simulink model "UAVmode"  (Simulink 8.3)
settings: Solver=ode45  StartTime=0.0  StopTime=20.0  RelTol=1e-3
values from neighbouring files (symbols this model uses):
  AngKD = UAV.AngKD    [UAVSimStart.m]
  AngKP = UAV.AngKP    [UAVSimStart.m]
  PosKD = UAV.PosKD    [UAVSimStart.m]
  PosKP = UAV.PosKP    [UAVSimStart.m]
  UAV = struct('Is',eye(3),'Is_inv',eye(3),'Mass',10,'L',1,'AllocationMoment',0,'RotorNum',0,'Type',[],'AllocationRotate',0,'GravityAcc',9.81,'Init_Pos',[0,0,0],'Init_Pos_Vel',[0,0,0],           'Course_ANG',0,'RWS',eye(3),'RSW',eye(3),'MaxTargetAng',[0,0,0],'MinTargetAng',[0,0,0],'TargetPos',[0,0,0],'TargetPos_Vel',[0,0,0],'LineTrack_ACC',[0,0,0],'LineTrack_Vel',[0,0,0],'CircleTrc_AngleACC',0.01,'CircleT ...(+517 chars)    [UAVSimStart.m]
libraries: fuzblock x3, simulink x2, aerolibtransform2 x2, vrlib x1
settings Model: Creator=Administrator  LastModifiedBy=jyl58
settings DataIOCC: SignalLoggingSaveFormat=Dataset
settings OptimizationCC: ExpressionDepthLimit=2147483647
settings DebuggingCC: FcnCallInpInsideContextMsg=EnableAllAsWarning
settings GRTTargetCC: CombineOutputUpdateFcns=on  GRTInterface=off

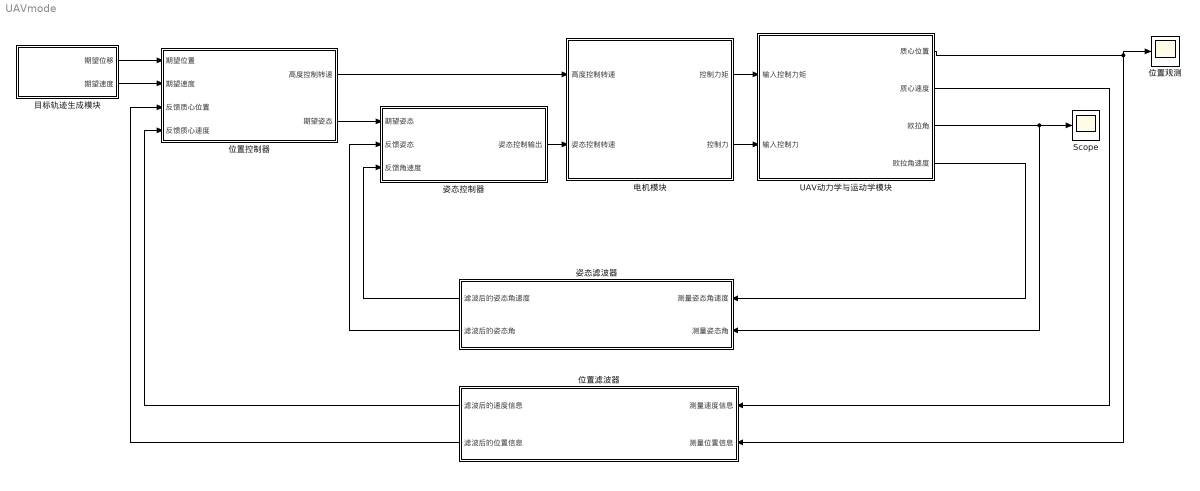
== system UAVmode ==
  Scope : Scope
      settings: YMin=-0.01  YMax=0.15
  UAV动力学与运动学模块 : Subsystem
  位置控制器 : Subsystem
  位置滤波器 : Subsystem
  位置观测 : Scope
      settings: YMin=-0.025  YMax=0.55  SaveName=ScopeData7
  姿态控制器 : Subsystem
  姿态滤波器 : Subsystem
  电机模块 : Subsystem
  目标轨迹生成模块 : Subsystem
  wires:
  电机模块/1(控制力矩) -> UAV动力学与运动学模块/1(输入控制力矩)
  姿态滤波器/2(滤波后的姿态角) -> 姿态控制器/2(反馈姿态)
  姿态滤波器/1(滤波后的姿态角速度) -> 姿态控制器/3(反馈角速度)
  电机模块/2(控制力) -> UAV动力学与运动学模块/2(输入控制力)
  UAV动力学与运动学模块/3(欧拉角) -> Scope/1, 姿态滤波器/2(测量姿态角)
  UAV动力学与运动学模块/4(欧拉角速度) -> 姿态滤波器/1(测量姿态角速度)
  UAV动力学与运动学模块/2(质心速度) -> 位置滤波器/1(测量速度信息)
  位置滤波器/1(滤波后的速度信息) -> 位置控制器/4(反馈质心速度)
  位置滤波器/2(滤波后的位置信息) -> 位置控制器/3(反馈质心位置)
  位置控制器/2(期望姿态) -> 姿态控制器/1(期望姿态)
  姿态控制器/1(姿态控制输出) -> 电机模块/2(姿态控制转速)
  目标轨迹生成模块/1(期望位移) -> 位置控制器/1(期望位置)
  目标轨迹生成模块/2(期望速度) -> 位置控制器/2(期望速度)
  位置控制器/1(高度控制转速) -> 电机模块/1(高度控制转速)
  UAV动力学与运动学模块/1(质心位置) -> 位置滤波器/2(测量位置信息), 位置观测/1

== system UAVmode/UAV动力学与运动学模块 ==
  输入控制力矩 : Inport
  输入控制力 : Inport  Port=2
  Terminator : Terminator
  姿态方程 : Subsystem
  质心运动方程 : Subsystem
  质心位置 : Outport
  质心速度 : Outport  Port=2
  欧拉角 : Outport  Port=3
  欧拉角速度 : Outport  Port=4
  wires:
  输入控制力矩/1 -> 姿态方程/1(控制力矩)
  姿态方程/2(欧拉角) -> 欧拉角/1, 质心运动方程/2(姿态角)
  姿态方程/3(欧拉角速度) -> 欧拉角速度/1
  输入控制力/1 -> 质心运动方程/1(控制力输入)
  质心运动方程/1(惯性系下质心位置) -> 质心位置/1
  质心运动方程/2(惯性系下速度) -> 质心速度/1
  姿态方程/1(惯性加速度) -> Terminator/1

== system UAVmode/位置控制器 ==
  期望位置 : Inport
  期望速度 : Inport  Port=2
  反馈质心位置 : Inport  Port=3
  反馈质心速度 : Inport  Port=4
  位置控制器 : Subsystem
  质心位置信息 : Subsystem
  高度控制转速 : Outport
  期望姿态 : Outport  Port=2
  wires:
  质心位置信息/1(位置偏差) -> 位置控制器/1(质心位置偏差)
  质心位置信息/2(速度偏差) -> 位置控制器/2(速度偏差)
  反馈质心位置/1 -> 质心位置信息/3(反馈质心位置)
  位置控制器/1(高度转速) -> 高度控制转速/1
  位置控制器/2(期望姿态) -> 期望姿态/1
  反馈质心速度/1 -> 质心位置信息/4(反馈质心速度)
  期望位置/1 -> 质心位置信息/1(期望位置)
  期望速度/1 -> 质心位置信息/2(期望速度)

== system UAVmode/位置滤波器 ==
  note: 暂不加滤波器
  note: 暂不加滤波器
  测量速度信息 : Inport
  测量位置信息 : Inport  Port=2
  滤波后的速度信息 : Outport
  滤波后的位置信息 : Outport  Port=2
  wires:
  测量位置信息/1 -> 滤波后的位置信息/1
  测量速度信息/1 -> 滤波后的速度信息/1

== system UAVmode/姿态控制器 ==
  期望姿态 : Inport
  反馈姿态 : Inport  Port=2
  反馈角速度 : Inport  Port=3
  姿态偏差信息 : Subsystem
  姿态控制器 : Subsystem
  期望角速度 : Constant  Value=UAV.TargetAng_Vel
  姿态控制输出 : Outport
  wires:
  反馈姿态/1 -> 姿态偏差信息/2(反馈姿态), 姿态控制器/4(反馈姿态)
  反馈角速度/1 -> 姿态偏差信息/4(反馈角速度), 姿态控制器/3(反馈角速度)
  期望角速度/1 -> 姿态偏差信息/3(期望角速度)
  期望姿态/1 -> 姿态偏差信息/1(期望姿态)
  姿态控制器/1(控制输出) -> 姿态控制输出/1
  姿态偏差信息/1(姿态角偏差) -> 姿态控制器/1(姿态角偏差)
  姿态偏差信息/2(姿态角速度偏差) -> 姿态控制器/2(角速度偏差)

== system UAVmode/姿态滤波器 ==
  note: 暂时不加滤波
  note: 暂时不加滤波
  测量姿态角速度 : Inport
  测量姿态角 : Inport  Port=2
  滤波后的姿态角速度 : Outport
  滤波后的姿态角 : Outport  Port=2
  wires:
  测量姿态角/1 -> 滤波后的姿态角/1
  测量姿态角速度/1 -> 滤波后的姿态角速度/1

== system UAVmode/电机模块 ==
  高度控制转速 : Inport
  姿态控制转速 : Inport  Port=2
  执行 : Subsystem
  转速融合 : Subsystem
  控制力矩 : Outport
  控制力 : Outport  Port=2
  wires:
  执行/1(控制力矩输出) -> 控制力矩/1
  执行/2(控制力输出) -> 控制力/1
  姿态控制转速/1 -> 转速融合/2(姿态控制转速)
  高度控制转速/1 -> 转速融合/1(高度控制转速)
  转速融合/1(电机总控制转速输出) -> 执行/1(控制转速)

== system UAVmode/目标轨迹生成模块 ==
  Constant : Constant  Value=0
  Constant1 : Constant  Value=0
  圆轨迹生成器 : Subsystem
  直线轨迹生成器 : Subsystem
  轨迹类型选择开关 : Constant  Value=UAV.TraceType
  轨迹选择器 : MultiPortSwitch
  轨迹选择器1 : MultiPortSwitch
  期望位移 : Outport
  期望速度 : Outport  Port=2
  wires:
  直线轨迹生成器/1(期望位置) -> 轨迹选择器/2
  圆轨迹生成器/1(期望位置) -> 轨迹选择器/3
  轨迹选择器1/1 -> 期望速度/1
  圆轨迹生成器/2(期望速度) -> 轨迹选择器1/3
  直线轨迹生成器/2(期望速度) -> 轨迹选择器1/2
  轨迹类型选择开关/1 -> 轨迹选择器1/1, 轨迹选择器/1
  Constant/1 -> 轨迹选择器/4
  Constant1/1 -> 轨迹选择器1/4
  轨迹选择器/1 -> 期望位移/1

== system UAVmode/UAV动力学与运动学模块/姿态方程 ==
  控制力矩 : Inport
  Sum : Sum  Inputs=|++
  姿态动力学方程 : Subsystem
  姿态运动学 : Subsystem
  干扰生成模块 : Subsystem
  惯性加速度 : Outport
  欧拉角 : Outport  Port=2
  欧拉角速度 : Outport  Port=3
  wires:
  姿态动力学方程/1(惯性角速度) -> 姿态运动学/1(Wbi), 惯性加速度/1
  姿态运动学/1(欧拉角) -> 欧拉角/1
  姿态运动学/2(欧拉角速度) -> 欧拉角速度/1
  控制力矩/1 -> Sum/1
  Sum/1 -> 姿态动力学方程/1(输入力矩)
  干扰生成模块/1(干扰输出) -> Sum/2

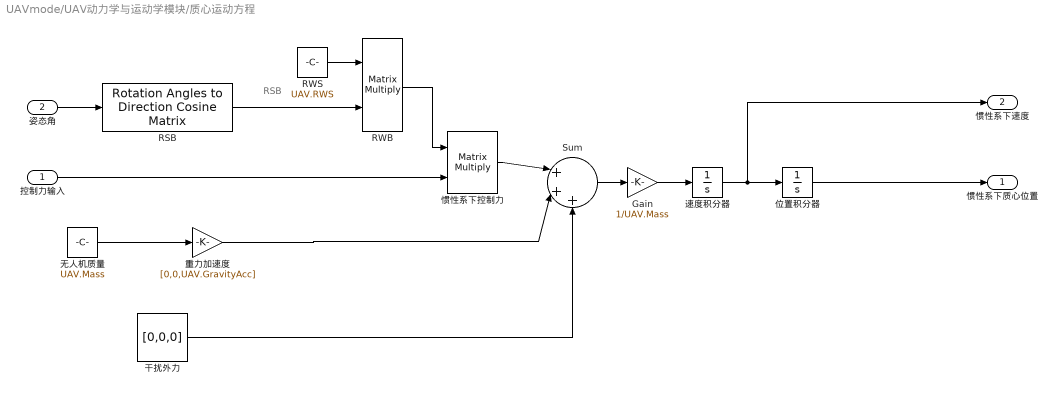
== system UAVmode/UAV动力学与运动学模块/质心运动方程 ==
  note: RSB
  控制力输入 : Inport
  姿态角 : Inport  Port=2
  Gain : Gain  Gain=1/UAV.Mass
  RSB : aerolibtransform2/Rotation Angles to Direction Cosine Matrix  rotationOrder=XYZ
  RWB : Product  Multiplication=Matrix(*)  RndMeth=Zero
  RWS : Constant  Value=UAV.RWS
  Sum : Sum  Inputs=|+++
  位置积分器 : Integrator  InitialCondition=UAV.Init_Pos
  干扰外力 : Constant  Value=[0,0,0]
  惯性系下控制力 : Product  Multiplication=Matrix(*)  RndMeth=Zero
  无人机质量 : Constant  Value=UAV.Mass
  速度积分器 : Integrator  InitialCondition=[0,0,0]
  重力加速度 : Gain  Gain=[0,0,UAV.GravityAcc]
  惯性系下质心位置 : Outport
  惯性系下速度 : Outport  Port=2
  wires:
  无人机质量/1 -> 重力加速度/1
  重力加速度/1 -> Sum/2
  速度积分器/1 -> 位置积分器/1, 惯性系下速度/1
  位置积分器/1 -> 惯性系下质心位置/1
  控制力输入/1 -> 惯性系下控制力/2
  惯性系下控制力/1 -> Sum/1
  干扰外力/1 -> Sum/3
  姿态角/1 -> RSB/1
  RSB/1 -> RWB/2
  RWS/1 -> RWB/1
  RWB/1 -> 惯性系下控制力/1
  Gain/1 -> 速度积分器/1
  Sum/1 -> Gain/1

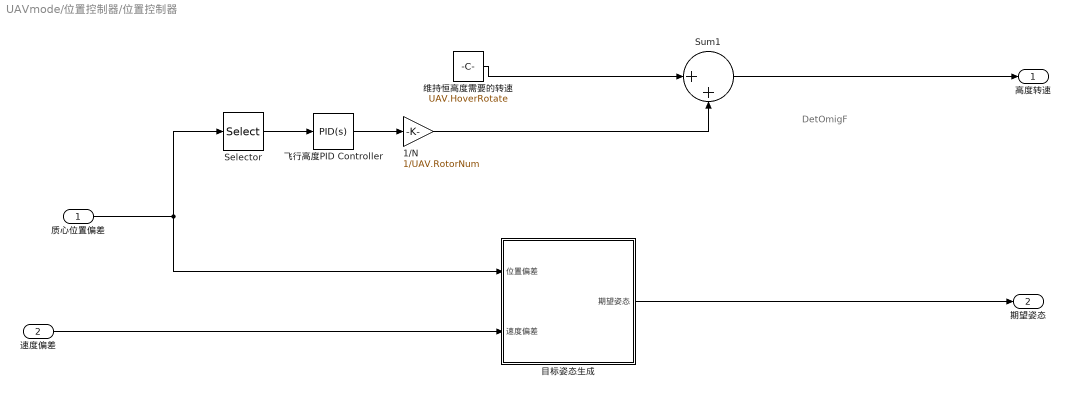
== system UAVmode/位置控制器/位置控制器 ==
  note: DetOmigF
  质心位置偏差 : Inport
  速度偏差 : Inport  Port=2
  1/N : Gain  Gain=1/UAV.RotorNum
  Selector : Selector  InputPortWidth=3  Indices=[3]
  Sum1 : Sum  Inputs=|++
  目标姿态生成 : Subsystem
  维持恒高度需要的转速 : Constant  Value=UAV.HoverRotate
  飞行高度PID Controller : simulink/Continuous/PID Controller  Controller=PID  TimeDomain=Continuous-time  SampleTime=1  IntegratorMethod=Forward Euler  FilterMethod=Forward Euler  Form=Parallel  P=-UAV.AltKP  I=-UAV.AltKI  D=-UAV.AltKD  N=1  InitialConditionSource=internal  InitialConditionForIntegrator=0  InitialConditionForFilter=0  ExternalReset=none  LimitOutput=off  UpperSaturationLimit=inf  LowerSaturationLimit=-inf  LinearizeAsGain=off  AntiWindupMode=none  Kb=1  TrackingMode=off  Kt=1  PParamMin=[]  PParamMax=[]  IParamMin=[]  IParamMax=[]  DParamMin=[]  DParamMax=[]  NParamMin=[]  NParamMax=[]  KbParamMin=[]  KbParamMax=[]  KtParamMin=[]  KtParamMax=[]  POutMin=[]  POutMax=[]  IOutMin=[]  IOutMax=[]  DOutMin=[]  DOutMax=[]  NOutMin=[]  NOutMax=[]  KbOutMin=[]  KbOutMax=[]  KtOutMin=[]  KtOutMax=[]  IntegratorOutMin=[]  IntegratorOutMax=[]  FilterOutMin=[]  FilterOutMax=[]  SumOutMin=[]  SumOutMax=[]  SumI1OutMin=[]  SumI1OutMax=[]  SumI2OutMin=[]  SumI2OutMax=[]  SumI3OutMin=[]  SumI3OutMax=[]  SumDOutMin=[]  SumDOutMax=[]  SaturationOutMin=[]  SaturationOutMax=[]  IntegratorContinuousStateAttributes=''  IntegratorStateMustResolveToSignalObject=off  IntegratorRTWStateStorageClass=Auto  FilterContinuousStateAttributes=''  FilterStateMustResolveToSignalObject=off  FilterRTWStateStorageClass=Auto
  高度转速 : Outport
  期望姿态 : Outport  Port=2
  wires:
  目标姿态生成/1(期望姿态) -> 期望姿态/1
  Sum1/1 -> 高度转速/1
  维持恒高度需要的转速/1 -> Sum1/1
  质心位置偏差/1 -> 目标姿态生成/1(位置偏差), Selector/1
  速度偏差/1 -> 目标姿态生成/2(速度偏差)
  飞行高度PID Controller/1 -> 1/N/1
  1/N/1 -> Sum1/2
  Selector/1 -> 飞行高度PID Controller/1

== system UAVmode/位置控制器/质心位置信息 ==
  期望位置 : Inport
  期望速度 : Inport  Port=2
  反馈质心位置 : Inport  Port=3
  反馈质心速度 : Inport  Port=4
  Sum : Sum  Inputs=|+-
  Sum1 : Sum  Inputs=|+-
  位置偏差 : Outport
  速度偏差 : Outport  Port=2
  wires:
  反馈质心位置/1 -> Sum/2
  反馈质心速度/1 -> Sum1/2
  Sum/1 -> 位置偏差/1
  Sum1/1 -> 速度偏差/1
  期望位置/1 -> Sum/1
  期望速度/1 -> Sum1/1

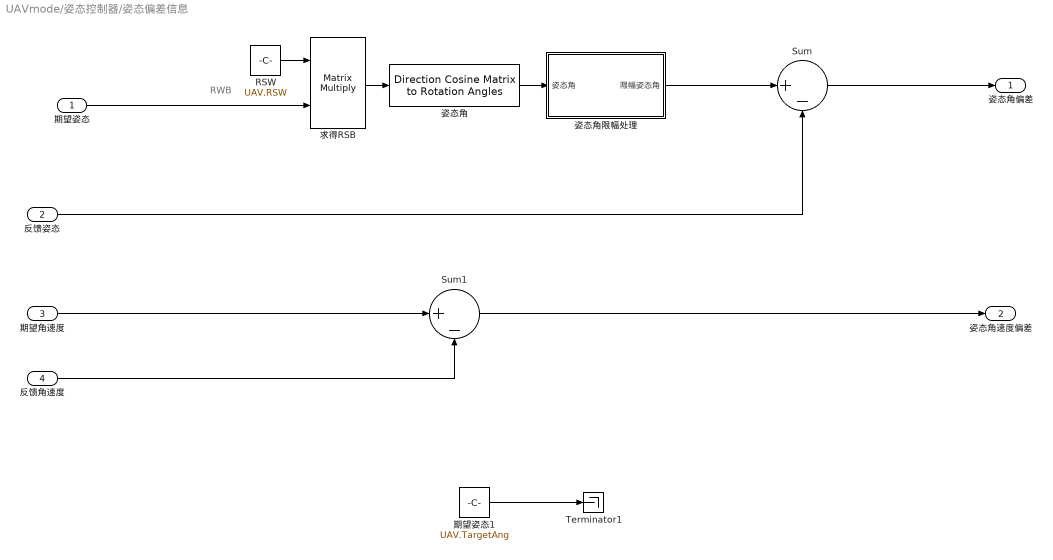
== system UAVmode/姿态控制器/姿态偏差信息 ==
  note: RWB
  期望姿态 : Inport
  反馈姿态 : Inport  Port=2
  期望角速度 : Inport  Port=3
  反馈角速度 : Inport  Port=4
  RSW : Constant  Value=UAV.RSW
  Sum : Sum  Inputs=|+-
  Sum1 : Sum  Inputs=|+-
  Terminator1 : Terminator
  姿态角 : aerolibtransform2/Direction Cosine Matrix to Rotation Angles  rotationOrder=XYZ  lim=Default
      settings: AttributesFormatString=Rotation Order: %<rotationOrder>
  姿态角限幅处理 : Subsystem
  期望姿态1 : Constant  Value=UAV.TargetAng
  求得RSB : Product  Multiplication=Matrix(*)  RndMeth=Zero
  姿态角偏差 : Outport
  姿态角速度偏差 : Outport  Port=2
  wires:
  反馈角速度/1 -> Sum1/2
  Sum/1 -> 姿态角偏差/1
  Sum1/1 -> 姿态角速度偏差/1
  反馈姿态/1 -> Sum/2
  期望角速度/1 -> Sum1/1
  求得RSB/1 -> 姿态角/1
  RSW/1 -> 求得RSB/1
  姿态角/1 -> 姿态角限幅处理/1(姿态角)
  期望姿态1/1 -> Terminator1/1
  期望姿态/1 -> 求得RSB/2
  姿态角限幅处理/1(限幅姿态角) -> Sum/1

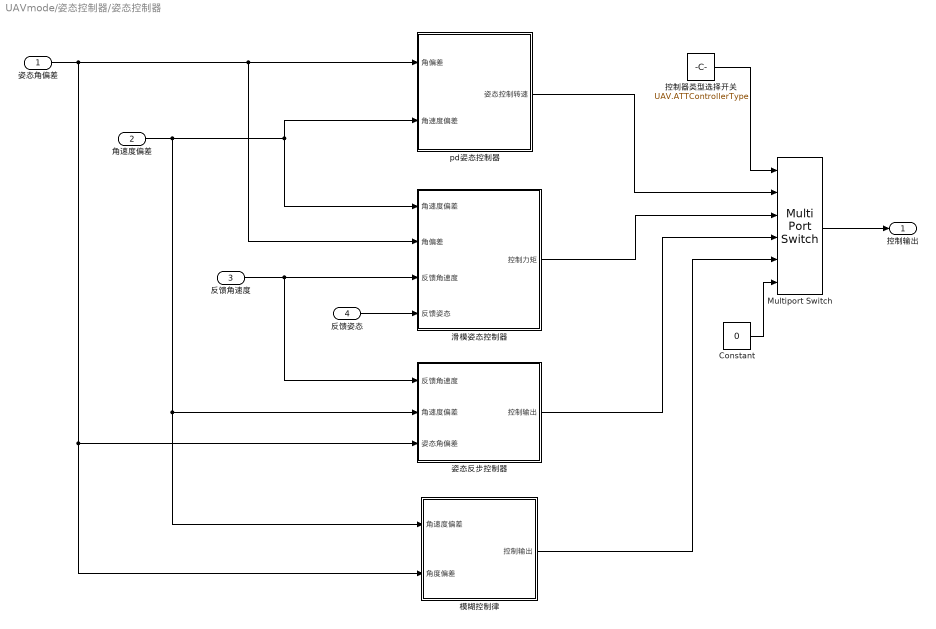
== system UAVmode/姿态控制器/姿态控制器 ==
  姿态角偏差 : Inport
  角速度偏差 : Inport  Port=2
  反馈角速度 : Inport  Port=3
  反馈姿态 : Inport  Port=4
  Constant : Constant  Value=0
  Multiport Switch : MultiPortSwitch  Inputs=5
  pd姿态控制器 : Subsystem
  姿态反步控制器 : Subsystem
  控制器类型选择开关 : Constant  Value=UAV.ATTControllerType
  模糊控制律 : Subsystem
  滑模姿态控制器 : Subsystem
  控制输出 : Outport
  wires:
  姿态角偏差/1 -> 滑模姿态控制器/2(角偏差), pd姿态控制器/1(角偏差), 模糊控制律/2(角度偏差), 姿态反步控制器/3(姿态角偏差)
  角速度偏差/1 -> 滑模姿态控制器/1(角速度偏差), pd姿态控制器/2(角速度偏差), 模糊控制律/1(角速度偏差), 姿态反步控制器/2(角速度偏差)
  pd姿态控制器/1(姿态控制转速) -> Multiport Switch/2
  反馈角速度/1 -> 姿态反步控制器/1(反馈角速度), 滑模姿态控制器/3(反馈角速度)
  反馈姿态/1 -> 滑模姿态控制器/4(反馈姿态)
  Multiport Switch/1 -> 控制输出/1
  滑模姿态控制器/1(控制力矩) -> Multiport Switch/3
  控制器类型选择开关/1 -> Multiport Switch/1
  姿态反步控制器/1(控制输出) -> Multiport Switch/4
  Constant/1 -> Multiport Switch/6
  模糊控制律/1(控制输出) -> Multiport Switch/5

== system UAVmode/电机模块/执行 ==
  note: 每个电机输出的作用力
  note: 电机输出作用力和
  控制转速 : Inport
  体坐标系下的总作用力 : MATLAB Function  TreatAsAtomicUnit=on
  力臂与力矩分配矩阵 : Constant  Value=UAV.AllocationMoment
  生成控制力矩 : Product  Multiplication=Matrix(*)  RndMeth=Zero
  电机系数 : Gain  Gain=UAV.RotorKF
  转速平方 : MATLAB Function  TreatAsAtomicUnit=on
  控制力矩输出 : Outport
  控制力输出 : Outport  Port=2
  wires:
  力臂与力矩分配矩阵/1 -> 生成控制力矩/1
  生成控制力矩/1 -> 控制力矩输出/1
  电机系数/1 -> 生成控制力矩/2, 体坐标系下的总作用力/1(u)
  控制转速/1 -> 转速平方/1(u)
  转速平方/1(y) -> 电机系数/1
  体坐标系下的总作用力/1(y) -> 控制力输出/1

== system UAVmode/电机模块/转速融合 ==
  note: 电机姿态控制转速输出
  高度控制转速 : Inport
  姿态控制转速 : Inport  Port=2
  Gain : Gain  Gain=ones(1,UAV.RotorNum)
  Mux : Mux  Inputs=2
  Product : Product  Multiplication=Matrix(*)  RndMeth=Zero
  电机转速分配矩阵 : Constant  Value=UAV.AllocationRotate
  转速融合 : MATLAB Function  TreatAsAtomicUnit=on
  电机总控制转速输出 : Outport
  wires:
  转速融合/1(y) -> 电机总控制转速输出/1
  Gain/1 -> Mux/2
  高度控制转速/1 -> Gain/1
  电机转速分配矩阵/1 -> Product/1
  姿态控制转速/1 -> Product/2
  Product/1 -> Mux/1
  Mux/1 -> 转速融合/1(u)

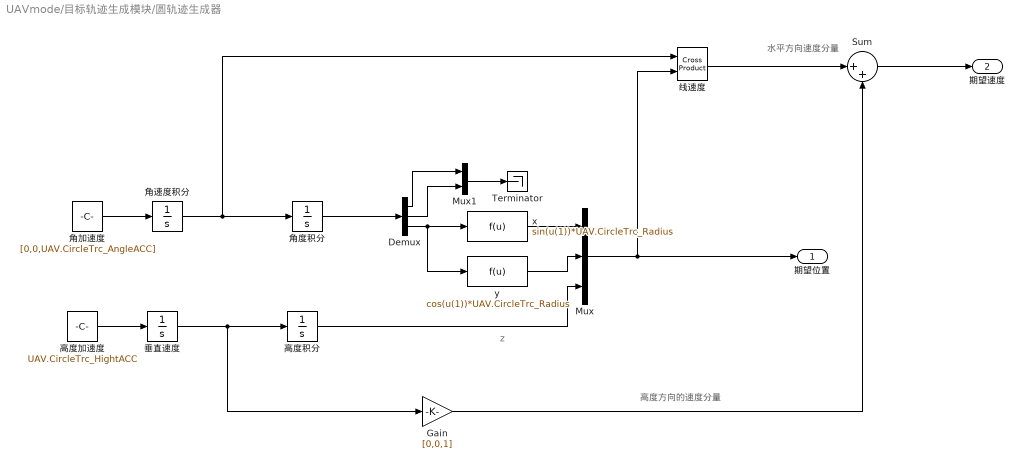
== system UAVmode/目标轨迹生成模块/圆轨迹生成器 ==
  note: z
  note: 高度方向的速度分量
  note: 水平方向速度分量
  Demux : Demux  Outputs=3
  Gain : Gain  Gain=[0,0,1]
  Mux : Mux  Inputs=3
  Mux1 : Mux  Inputs=2
  Sum : Sum  Inputs=|++
  Terminator : Terminator
  x : Fcn  Expr=sin(u(1))*UAV.CircleTrc_Radius
  y : Fcn  Expr=cos(u(1))*UAV.CircleTrc_Radius
  垂直速度 : Integrator
  线速度 : vrlib/Utilities/Cross Product
  角加速度 : Constant  Value=[0,0,UAV.CircleTrc_AngleACC]
  角度积分 : Integrator
  角速度积分 : Integrator  InitialCondition=[0,0,0.01]
  高度加速度 : Constant  Value=UAV.CircleTrc_HightACC
  高度积分 : Integrator
  期望位置 : Outport
  期望速度 : Outport  Port=2
  wires:
  角加速度/1 -> 角速度积分/1
  角速度积分/1 -> 角度积分/1, 线速度/1
  x/1 -> Mux/1
  y/1 -> Mux/2
  Mux/1 -> 期望位置/1, 线速度/2
  高度加速度/1 -> 垂直速度/1
  垂直速度/1 -> 高度积分/1, Gain/1
  高度积分/1 -> Mux/3
  角度积分/1 -> Demux/1
  Demux/3 -> x/1, y/1
  线速度/1 -> Sum/1
  Gain/1 -> Sum/2
  Sum/1 -> 期望速度/1
  Demux/1 -> Mux1/1
  Demux/2 -> Mux1/2
  Mux1/1 -> Terminator/1

== system UAVmode/目标轨迹生成模块/直线轨迹生成器 ==
  位移积分器 : Integrator  InitialCondition=[0,0,0]
  加速度 : Constant  Value=UAV.LineTrack_ACC
  速度积分器 : Integrator  InitialCondition=UAV.LineTrack_Vel
  期望位置 : Outport
  期望速度 : Outport  Port=2
  wires:
  加速度/1 -> 速度积分器/1
  速度积分器/1 -> 位移积分器/1, 期望速度/1
  位移积分器/1 -> 期望位置/1

== system UAVmode/UAV动力学与运动学模块/姿态方程/姿态动力学方程 ==
  note: omega
  输入力矩 : Inport
  "   " : Subsystem
  Integrator : Integrator  InitialCondition=[0;0;0]
  Matrix Gain : Gain  Gain=UAV.Is_inv  Multiplication=Matrix(K*u)  SaturateOnIntegerOverflow=on  OutDataTypeStr=Inherit: Same as input  ParamDataTypeStr=Inherit: Same as input
  Sum2 : Sum  Inputs=|-+
  惯性角速度 : Outport
  wires:
  Matrix Gain/1 -> Integrator/1
  Sum2/1 -> Matrix Gain/1
  "   "/1(Out1) -> Sum2/1
  Integrator/1 -> "   "/1(Wbi), 惯性角速度/1
  输入力矩/1 -> Sum2/2

== system UAVmode/UAV动力学与运动学模块/姿态方程/姿态运动学 ==
  note: 姿态角速度
  note: 姿态角
  note: Pothe
  note: Theta
  note: Fai
  Wbi : Inport
  Integrator : Integrator
  Integrator1 : Integrator
  Integrator2 : Integrator
  Mux1 : Mux  Inputs=3
  Mux2 : Mux  Inputs=3
  Subsystem1 : Subsystem
  欧拉角 : Outport
  欧拉角速度 : Outport  Port=2
  wires:
  Mux2/1 -> 欧拉角速度/1
  Subsystem1/2(Out2) -> Mux2/2, Integrator1/1
  Subsystem1/3(Out3) -> Mux2/3, Integrator2/1
  Subsystem1/1(Out1) -> Mux2/1, Integrator/1
  Mux1/1 -> Subsystem1/2(In2), 欧拉角/1
  Integrator2/1 -> Mux1/3
  Integrator1/1 -> Mux1/2
  Integrator/1 -> Mux1/1
  Wbi/1 -> Subsystem1/1(In1)

== system UAVmode/UAV动力学与运动学模块/姿态方程/干扰生成模块 ==
  Band-Limited White Noise : simulink/Sources/Band-Limited White Noise  Cov=[1]  Ts=0.1  seed=[23341]
  Gain : Gain  Gain=[1;1;1]
  干扰输出 : Outport
  wires:
  Band-Limited White Noise/1 -> Gain/1
  Gain/1 -> 干扰输出/1

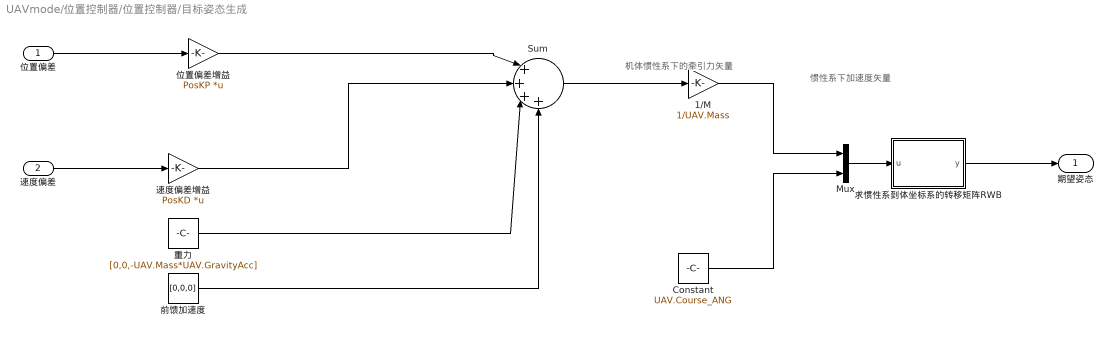
== system UAVmode/位置控制器/位置控制器/目标姿态生成 ==
  note: 机体惯性系下的牵引力矢量
  note: 惯性系下加速度矢量
  位置偏差 : Inport
  速度偏差 : Inport  Port=2
  1/M : Gain  Gain=1/UAV.Mass
  Constant : Constant  Value=UAV.Course_ANG
  Mux : Mux  Inputs=2
  Sum : Sum  Inputs=|++++
  位置偏差增益 : Gain  Gain=PosKP  Multiplication=Matrix(K*u)
  前馈加速度 : Constant  Value=[0,0,0]
  求惯性系到体坐标系的转移矩阵RWB : MATLAB Function  TreatAsAtomicUnit=on
  速度偏差增益 : Gain  Gain=PosKD  Multiplication=Matrix(K*u)
  重力 : Constant  Value=[0,0,-UAV.Mass*UAV.GravityAcc]
  期望姿态 : Outport
  wires:
  位置偏差/1 -> 位置偏差增益/1
  速度偏差/1 -> 速度偏差增益/1
  Sum/1 -> 1/M/1
  求惯性系到体坐标系的转移矩阵RWB/1(y) -> 期望姿态/1
  位置偏差增益/1 -> Sum/1
  速度偏差增益/1 -> Sum/2
  重力/1 -> Sum/3
  前馈加速度/1 -> Sum/4
  1/M/1 -> Mux/1
  Constant/1 -> Mux/2
  Mux/1 -> 求惯性系到体坐标系的转移矩阵RWB/1(u)

== system UAVmode/姿态控制器/姿态偏差信息/姿态角限幅处理 ==
  姿态角 : Inport
  Demux : Demux  Outputs=3
  Mux : Mux  Inputs=3
  俯仰角限幅 : Saturate  UpperLimit=UAV.MaxTargetAng(2)  LowerLimit=UAV.MinTargetAng(2)
  偏航角限幅 : Saturate  UpperLimit=UAV.MaxTargetAng(3)  LowerLimit=UAV.MinTargetAng(3)
  滚转角限幅 : Saturate  UpperLimit=UAV.MaxTargetAng(1)  LowerLimit=UAV.MinTargetAng(1)
  限幅姿态角 : Outport
  wires:
  姿态角/1 -> Demux/1
  Demux/2 -> 俯仰角限幅/1
  俯仰角限幅/1 -> Mux/2
  Demux/1 -> 滚转角限幅/1
  滚转角限幅/1 -> Mux/1
  Demux/3 -> 偏航角限幅/1
  偏航角限幅/1 -> Mux/3
  Mux/1 -> 限幅姿态角/1

== system UAVmode/姿态控制器/姿态控制器/pd姿态控制器 ==
  角偏差 : Inport
  角速度偏差 : Inport  Port=2
  KD : Gain  Gain=AngKD  Multiplication=Matrix(K*u)
  KP : Gain  Gain=AngKP  Multiplication=Matrix(K*u)
  Sum : Sum  Inputs=|++
  姿态控制转速 : Outport
  wires:
  角偏差/1 -> KP/1
  角速度偏差/1 -> KD/1
  KP/1 -> Sum/1
  KD/1 -> Sum/2
  Sum/1 -> 姿态控制转速/1

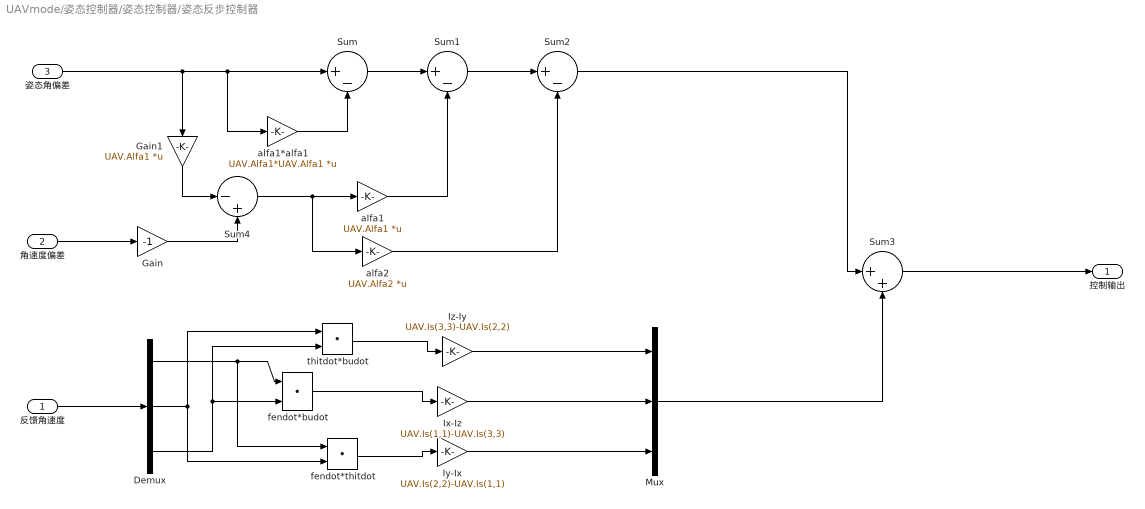
== system UAVmode/姿态控制器/姿态控制器/姿态反步控制器 ==
  反馈角速度 : Inport
  角速度偏差 : Inport  Port=2
  姿态角偏差 : Inport  Port=3
  Demux : Demux  Outputs=3
  Gain : Gain  Gain=-1
  Gain1 : Gain  Gain=UAV.Alfa1  Multiplication=Matrix(K*u)
  Ix-Iz : Gain  Gain=UAV.Is(1,1)-UAV.Is(3,3)
  Iy-Ix : Gain  Gain=UAV.Is(2,2)-UAV.Is(1,1)
  Iz-Iy : Gain  Gain=UAV.Is(3,3)-UAV.Is(2,2)
  Mux : Mux  Inputs=3
  Sum : Sum  Inputs=|+-
  Sum1 : Sum  Inputs=|+-
  Sum2 : Sum  Inputs=|+-
  Sum3 : Sum  Inputs=|++
  Sum4 : Sum  Inputs=|-+
  alfa1 : Gain  Gain=UAV.Alfa1  Multiplication=Matrix(K*u)
  alfa1*alfa1 : Gain  Gain=UAV.Alfa1*UAV.Alfa1  Multiplication=Matrix(K*u) (u vector)
  alfa2 : Gain  Gain=UAV.Alfa2  Multiplication=Matrix(K*u)
  fendot*budot : DotProduct  InputSameDT=on  OutDataTypeStr=Inherit: Inherit via internal rule
  fendot*thitdot : DotProduct  InputSameDT=on  OutDataTypeStr=Inherit: Inherit via internal rule
  thitdot*budot : DotProduct  InputSameDT=on  OutDataTypeStr=Inherit: Inherit via internal rule
  控制输出 : Outport
  wires:
  Sum3/1 -> 控制输出/1
  姿态角偏差/1 -> Sum/1, alfa1*alfa1/1, Gain1/1
  alfa1*alfa1/1 -> Sum/2
  Sum/1 -> Sum1/1
  alfa1/1 -> Sum1/2
  Sum1/1 -> Sum2/1
  alfa2/1 -> Sum2/2
  反馈角速度/1 -> Demux/1
  Mux/1 -> Sum3/2
  Demux/2 -> thitdot*budot/1, fendot*thitdot/2
  Demux/3 -> fendot*budot/2, thitdot*budot/2
  thitdot*budot/1 -> Iz-Iy/1
  Iz-Iy/1 -> Mux/1
  fendot*budot/1 -> Ix-Iz/1
  Ix-Iz/1 -> Mux/2
  Demux/1 -> fendot*thitdot/1, fendot*budot/1
  fendot*thitdot/1 -> Iy-Ix/1
  Iy-Ix/1 -> Mux/3
  Sum2/1 -> Sum3/1
  角速度偏差/1 -> Gain/1
  Sum4/1 -> alfa1/1, alfa2/1
  Gain/1 -> Sum4/2
  Gain1/1 -> Sum4/1

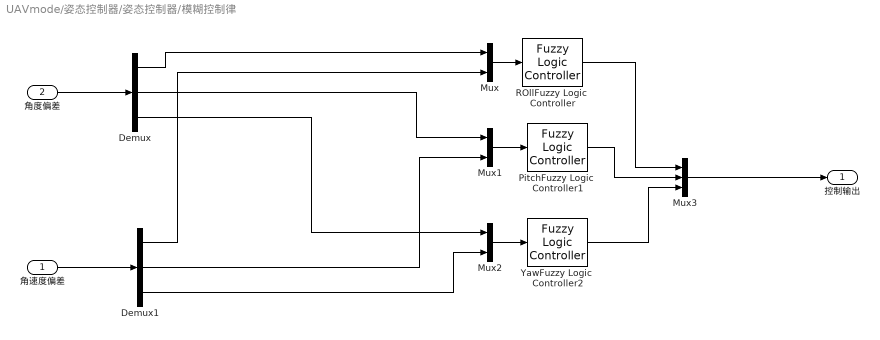
== system UAVmode/姿态控制器/姿态控制器/模糊控制律 ==
  角速度偏差 : Inport
  角度偏差 : Inport  Port=2
  Demux : Demux  Outputs=3
  Demux1 : Demux  Outputs=3
  Mux : Mux  Inputs=2
  Mux1 : Mux  Inputs=2
  Mux2 : Mux  Inputs=2
  Mux3 : Mux  Inputs=3
  PitchFuzzy Logic  Controller1 : fuzblock/Fuzzy Logic  Controller  fis='TESTFUZZY2.fis'
  ROllFuzzy Logic  Controller : fuzblock/Fuzzy Logic  Controller  fis='TESTFUZZY2.fis'
  YawFuzzy Logic  Controller2 : fuzblock/Fuzzy Logic  Controller  fis='TESTFUZZY2.fis'
  控制输出 : Outport
  wires:
  Mux3/1 -> 控制输出/1
  角度偏差/1 -> Demux/1
  角速度偏差/1 -> Demux1/1
  Mux/1 -> ROllFuzzy Logic  Controller/1
  Demux/2 -> Mux1/1
  Mux1/1 -> PitchFuzzy Logic  Controller1/1
  Mux2/1 -> YawFuzzy Logic  Controller2/1
  Demux/1 -> Mux/1
  Demux1/1 -> Mux/2
  Demux1/2 -> Mux1/2
  Demux/3 -> Mux2/1
  Demux1/3 -> Mux2/2
  ROllFuzzy Logic  Controller/1 -> Mux3/1
  PitchFuzzy Logic  Controller1/1 -> Mux3/2
  YawFuzzy Logic  Controller2/1 -> Mux3/3

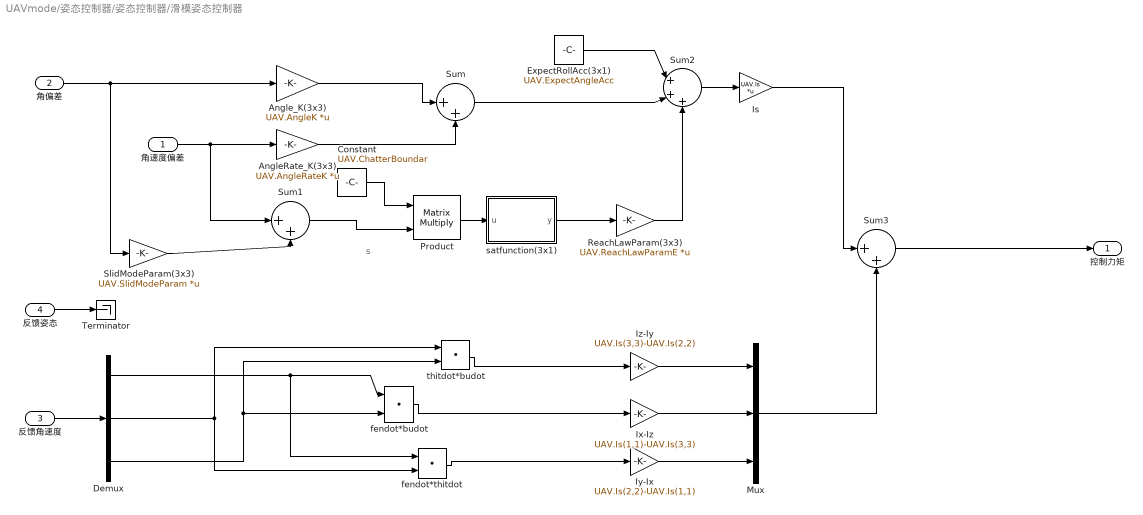
== system UAVmode/姿态控制器/姿态控制器/滑模姿态控制器 ==
  note: s
  角速度偏差 : Inport
  角偏差 : Inport  Port=2
  反馈角速度 : Inport  Port=3
  反馈姿态 : Inport  Port=4
  AngleRate_K(3x3) : Gain  Gain=UAV.AngleRateK  Multiplication=Matrix(K*u)
  Angle_K(3x3) : Gain  Gain=UAV.AngleK  Multiplication=Matrix(K*u)
  Constant : Constant  Value=UAV.ChatterBoundar
  Demux : Demux  Outputs=3
  ExpectRollAcc(3x1) : Constant  Value=UAV.ExpectAngleAcc
  Is : Gain  Gain=UAV.Is  Multiplication=Matrix(K*u)
  Ix-Iz : Gain  Gain=UAV.Is(1,1)-UAV.Is(3,3)
  Iy-Ix : Gain  Gain=UAV.Is(2,2)-UAV.Is(1,1)
  Iz-Iy : Gain  Gain=UAV.Is(3,3)-UAV.Is(2,2)
  Mux : Mux  Inputs=3
  Product : Product  Multiplication=Matrix(*)  RndMeth=Zero
  ReachLawParam(3x3) : Gain  Gain=UAV.ReachLawParamE  Multiplication=Matrix(K*u)
  SlidModeParam(3x3) : Gain  Gain=UAV.SlidModeParam  Multiplication=Matrix(K*u)
  Sum : Sum  Inputs=|++
  Sum1 : Sum  Inputs=|++
  Sum2 : Sum  Inputs=|+++
  Sum3 : Sum  Inputs=|++
  Terminator : Terminator
  fendot*budot : DotProduct  InputSameDT=on  OutDataTypeStr=Inherit: Inherit via internal rule
  fendot*thitdot : DotProduct  InputSameDT=on  OutDataTypeStr=Inherit: Inherit via internal rule
  satfunction(3x1) : MATLAB Function  TreatAsAtomicUnit=on
  thitdot*budot : DotProduct  InputSameDT=on  OutDataTypeStr=Inherit: Inherit via internal rule
  控制力矩 : Outport
  wires:
  角偏差/1 -> SlidModeParam(3x3)/1, Angle_K(3x3)/1
  角速度偏差/1 -> Sum1/1, AngleRate_K(3x3)/1
  AngleRate_K(3x3)/1 -> Sum/2
  Angle_K(3x3)/1 -> Sum/1
  SlidModeParam(3x3)/1 -> Sum1/2
  反馈姿态/1 -> Terminator/1
  Product/1 -> satfunction(3x1)/1(u)
  satfunction(3x1)/1(y) -> ReachLawParam(3x3)/1
  ReachLawParam(3x3)/1 -> Sum2/3
  Sum/1 -> Sum2/2
  ExpectRollAcc(3x1)/1 -> Sum2/1
  Sum2/1 -> Is/1
  反馈角速度/1 -> Demux/1
  Is/1 -> Sum3/1
  Mux/1 -> Sum3/2
  Sum3/1 -> 控制力矩/1
  Demux/2 -> thitdot*budot/1, fendot*thitdot/2
  Demux/3 -> fendot*budot/2, thitdot*budot/2
  thitdot*budot/1 -> Iz-Iy/1
  Iz-Iy/1 -> Mux/1
  fendot*budot/1 -> Ix-Iz/1
  Ix-Iz/1 -> Mux/2
  Demux/1 -> fendot*thitdot/1, fendot*budot/1
  fendot*thitdot/1 -> Iy-Ix/1
  Iy-Ix/1 -> Mux/3
  Constant/1 -> Product/1
  Sum1/1 -> Product/2

== system UAVmode/UAV动力学与运动学模块/姿态方程/姿态动力学方程/    ==
  note: Omega
  note: H
  Wbi : Inport
  AXB : Subsystem
  Matrix Gain : Gain  Gain=UAV.Is  Multiplication=Matrix(K*u)  SaturateOnIntegerOverflow=on  OutDataTypeStr=Inherit: Same as input  ParamDataTypeStr=Inherit: Same as input
  Out1 : Outport
  wires:
  Matrix Gain/1 -> AXB/2(In2)
  Wbi/1 -> Matrix Gain/1, AXB/1(In1)
  AXB/1(Out1) -> Out1/1

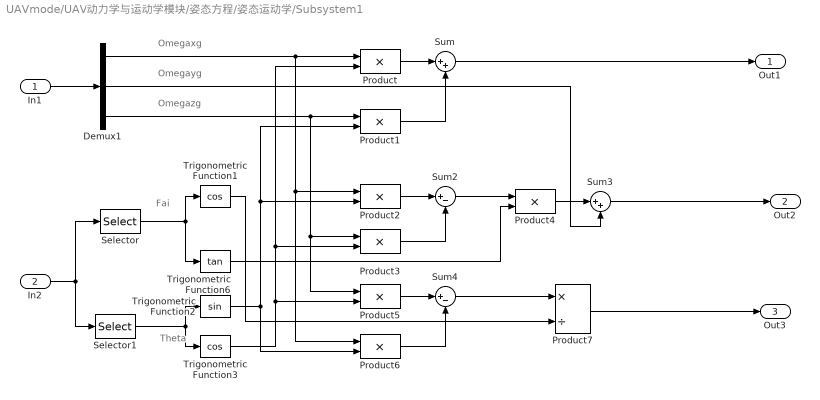
== system UAVmode/UAV动力学与运动学模块/姿态方程/姿态运动学/Subsystem1 ==
  note: Omegazg
  note: Omegayg
  note: Omegaxg
  note: Theta
  note: Fai
  In1 : Inport
  In2 : Inport  Port=2
  Demux1 : Demux  Outputs=3
  Product{,1..6} (7 alike) : Product  SaturateOnIntegerOverflow=on  InputSameDT=on  OutDataTypeStr=Inherit: Same as first input
  Product7 : Product  Inputs=*/  SaturateOnIntegerOverflow=on  OutDataTypeStr=Inherit: Same as first input
  Selector : Selector  InputPortWidth=3  Indices=[1]
  Selector1 : Selector  InputPortWidth=3  Indices=[2]
  Sum : Sum  Inputs=|++  SaturateOnIntegerOverflow=on  InputSameDT=on  OutDataTypeStr=Inherit: Same as first input
  Sum2 : Sum  Inputs=|+-  SaturateOnIntegerOverflow=on  InputSameDT=on  OutDataTypeStr=Inherit: Same as first input
  Sum3 : Sum  Inputs=|++  SaturateOnIntegerOverflow=on  InputSameDT=on  OutDataTypeStr=Inherit: Same as first input
  Sum4 : Sum  Inputs=|+-  SaturateOnIntegerOverflow=on  InputSameDT=on  OutDataTypeStr=Inherit: Same as first input
  Trigonometric Function1 : Trigonometry  Operator=cos
  Trigonometric Function2 : Trigonometry
  Trigonometric Function3 : Trigonometry  Operator=cos
  Trigonometric Function6 : Trigonometry  Operator=tan
  Out1 : Outport
  Out2 : Outport  Port=2
  Out3 : Outport  Port=3
  wires:
  Trigonometric Function1/1 -> Product7/2
  Sum4/1 -> Product7/1
  Demux1/2 -> Sum3/2
  Trigonometric Function6/1 -> Product4/2
  Trigonometric Function2/1 -> Product6/2, Product2/2, Product1/2
  Demux1/3 -> Product5/1, Product3/1, Product1/1
  Trigonometric Function3/1 -> Product5/2, Product3/2, Product/2
  Demux1/1 -> Product6/1, Product2/1, Product/1
  Product6/1 -> Sum4/2
  Product5/1 -> Sum4/1
  Product4/1 -> Sum3/1
  Sum2/1 -> Product4/1
  Product3/1 -> Sum2/2
  Product2/1 -> Sum2/1
  Sum/1 -> Out1/1
  Product1/1 -> Sum/2
  Product/1 -> Sum/1
  Selector1/1 -> Trigonometric Function3/1, Trigonometric Function2/1
  Selector/1 -> Trigonometric Function1/1, Trigonometric Function6/1
  In2/1 -> Selector1/1, Selector/1
  In1/1 -> Demux1/1
  Sum3/1 -> Out2/1
  Product7/1 -> Out3/1

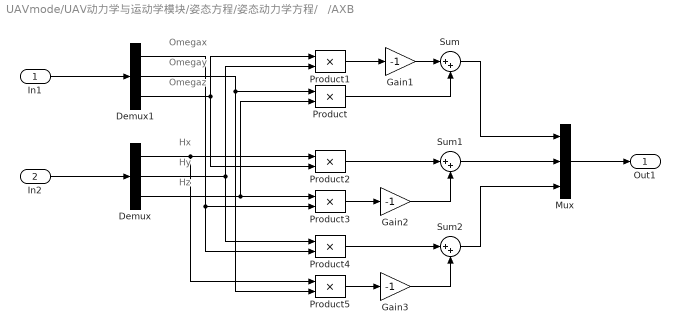
== system UAVmode/UAV动力学与运动学模块/姿态方程/姿态动力学方程/   /AXB ==
  note: Omegaz
  note: Omegay
  note: Omegax
  note: Hz
  note: Hy
  note: Hx
  In1 : Inport
  In2 : Inport  Port=2
  Demux : Demux  Outputs=3
  Demux1 : Demux  Outputs=3
  Gain1 : Gain  Gain=-1  SaturateOnIntegerOverflow=on  OutDataTypeStr=Inherit: Same as input  ParamDataTypeStr=Inherit: Same as input
  Gain2 : Gain  Gain=-1  SaturateOnIntegerOverflow=on  OutDataTypeStr=Inherit: Same as input  ParamDataTypeStr=Inherit: Same as input
  Gain3 : Gain  Gain=-1  SaturateOnIntegerOverflow=on  OutDataTypeStr=Inherit: Same as input  ParamDataTypeStr=Inherit: Same as input
  Mux : Mux  Inputs=3
  Product{,1..5} (6 alike) : Product  SaturateOnIntegerOverflow=on  InputSameDT=on  OutDataTypeStr=Inherit: Same as first input
  Sum : Sum  Inputs=|++  SaturateOnIntegerOverflow=on  InputSameDT=on  OutDataTypeStr=Inherit: Same as first input
  Sum1 : Sum  Inputs=|++  SaturateOnIntegerOverflow=on  InputSameDT=on  OutDataTypeStr=Inherit: Same as first input
  Sum2 : Sum  Inputs=|++  SaturateOnIntegerOverflow=on  InputSameDT=on  OutDataTypeStr=Inherit: Same as first input
  Out1 : Outport
  wires:
  In2/1 -> Demux/1
  Mux/1 -> Out1/1
  Sum2/1 -> Mux/3
  Sum1/1 -> Mux/2
  Demux1/3 -> Product2/2, Product1/1
  Demux1/2 -> Product5/2, Product/1
  Demux1/1 -> Product4/2, Product3/2
  Sum/1 -> Mux/1
  Gain3/1 -> Sum2/2
  Product4/1 -> Sum2/1
  Product5/1 -> Gain3/1
  Gain2/1 -> Sum1/2
  Product2/1 -> Sum1/1
  Product3/1 -> Gain2/1
  Product/1 -> Sum/2
  Gain1/1 -> Sum/1
  Product1/1 -> Gain1/1
  Demux/3 -> Product3/1, Product/2
  Demux/2 -> Product4/1, Product1/2
  Demux/1 -> Product5/1, Product2/1
  In1/1 -> Demux1/1

== matlab function 位置控制器/位置控制器/目标姿态生成/求惯性系到体坐标系的转移矩阵RWB ==
  data: u input double; y output double
function y = fcn(u)
%#codegen
% Xw=u(1);
% Yw=u(2);
% Zw=u(3);
ANG_course=u(4); % course angle
bu=ANG_course-pi/2;
ZBw=[u(1),u(2),u(3)]';
% To get the ZB from Acc 
% the body zB is 
ZW = -ZBw./norm(ZBw);
XC=[cos(ANG_course),sin(ANG_course),0]';  % 
YW=cross(ZW,XC);          % 
XW=cross(YW,ZW);
y=[XW,YW,ZW]; % rotation matrix

== matlab function 电机模块/执行/转速平方 ==
  data: u input double; y output double
function y = fcn(u)
%#codegen

switch(size(u,1))
    case 4
            y = [u(1)^2,u(2)^2,u(3)^2,u(4)^2]';
    case 6
            y = [u(1)^2,u(2)^2,u(3)^2,u(4)^2,u(5)^2,u(6)^2]';
    case 8
            y = [u(1)^2,u(2)^2,u(3)^2,u(4)^2,u(5)^2,u(6)^2,u(7)^2,u(8)^2]';
end

== matlab function 电机模块/执行/体坐标系下的总作用力 ==
  data: u input double; y output double
function y = fcn(u)
%#codegen
switch(size(u,1))
    case 4
        F= u(1)+u(2)+u(3)+u(4);
    case 6
        F= u(1)+u(2)+u(3)+u(4)+u(5)+u(6);
    case 8
        F= u(1)+u(2)+u(3)+u(4)+u(5)+u(6)+u(7)+u(8);
end
y=[0,0,-F]';

== matlab function 姿态控制器/姿态控制器/滑模姿态控制器/satfunction(3x1) ==
  data: u input double; y output double
function y = fcn(u)
%#codegen
s1=u(1);
s2=u(2);
s3=u(3);

if ((abs(s1))>1)
    y1=sign(s1);
else
    y1=s1;
end

if ((abs(s2))>1)
    y2=sign(s2);
else
    y2=s2;
end

if ((abs(s3))>1)
    y3=sign(s3);
else
    y3=s3;
end
y = [y1,y2,y3]';

%  y=sign(u);

== matlab function 电机模块/转速融合/转速融合 ==
  data: u input double; y output double
function y = fcn(u)
%#codegen
switch(size(u,1))
    case 8;
      AttiRotor=[u(1),u(2),u(3),u(4)]';
      AltRotor=[u(5),u(6),u(7),u(8)]';% all same
      AllRotor=AttiRotor+AltRotor; 
      MinRotor=min(AllRotor);
      if (MinRotor<0)
        Scale=AltRotor(1)/(AltRotor(1)-MinRotor);
        AttiRotor=Scale.*AttiRotor;
        AllRotor=AltRotor+AttiRotor;
      end
    case 12;
      AttiRotor=[u(1),u(2),u(3),u(4),u(5),u(6),]';
      AltRotor= [u(7),u(8),u(9),u(10),u(11),u(12)]';
      AllRotor=AttiRotor+AltRotor; 
      MinRotor=min(AllRotor);
      if (MinRotor<0)
        Scale=AltRotor(1)/(AltRotor(1)-MinRotor);
        AttiRotor=Scale.*AttiRotor;
        AllRotor=AltRotor+AttiRotor;
      end
    case 16;
      AttiRotor=[u(1),u(2),u(3),u(4),u(5),u(6),u(7),u(8)]';
      AltRotor= [u(9),u(10),u(11),u(12),u(13),u(14),u(5),u(16)]'; 
      AllRotor=AttiRotor+AltRotor; 
      MinRotor=min(AllRotor);
      if (MinRotor<0)
        Scale=AltRotor(1)/(AltRotor(1)-MinRotor);
        AttiRotor=Scale.*AttiRotor;
        AllRotor=AltRotor+AttiRotor;
      end
    otherwise
end
y = AllRotor;
